simulink model "SPARCS_MIL"  (R2024a)
settings: Solver=VariableStepAuto  StartTime=0.0  StopTime=10.0  RelTol=1e-3
undefined symbols (not defined in the file or in its folder): attitude, epoch, IAU, juliandate, km, m, om0_x, om0_y, om0_z, s, satellite, simulator, WMM2020
libraries: simulink_extras x16, sharedtransform x14, SepehrMILLib x10, aerolibconvert2 x9, matrix_library x3, simulink x3, aerolibutil x3, vrlib x2, aerolibgravity2 x2, aerolibtransform2 x2
(part 2 of 2)

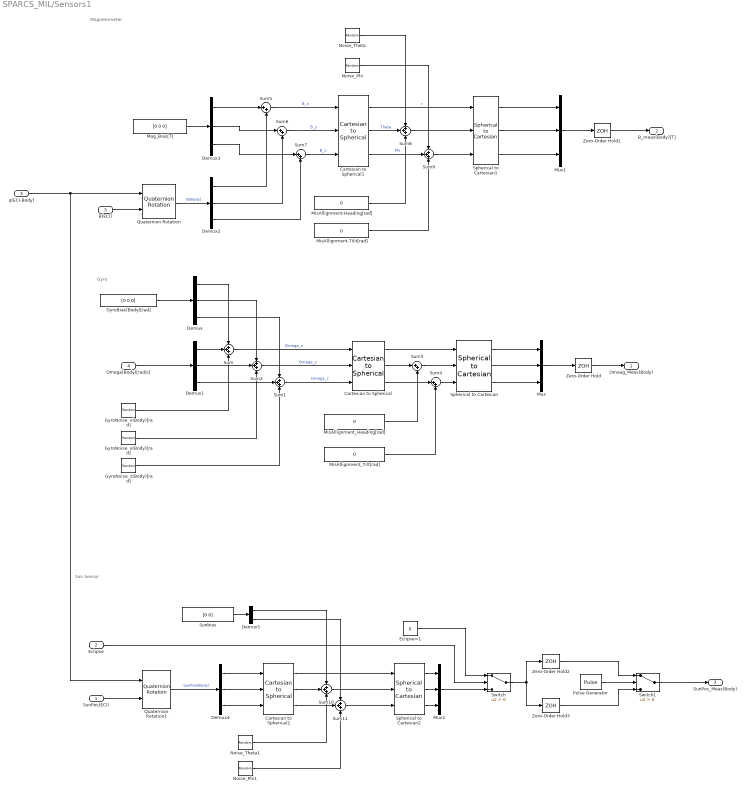
== system SPARCS_MIL/Sensors1 ==
  note: Magnetometer
  note: Sun Sensor
  note: Gyro
  SunPos(ECI) : Inport
  Eclipse : Inport  Port=2
  q(ECI-Body) : Inport  Port=3
  Omega(Body)[rad/s] : Inport  Port=4
  B(ECI) : InportShadow  Port=3
  Cartesian to Spherical : simulink_extras/Transformations/Cartesian to Spherical
  Cartesian to Spherical1 : simulink_extras/Transformations/Cartesian to Spherical
  Cartesian to Spherical2 : simulink_extras/Transformations/Cartesian to Spherical
  Demux{,1..4} (5 alike) : Demux  Outputs=3
  Demux5 : Demux  Outputs=2
  Eclipse=1 : Constant  Value=0
  GyroBias(Body)[rad] : Constant  Value=[0 0 0]
  GyroNoise_x(Body)[rad] : RandomNumber  SampleTime=0.1
  GyroNoise_y(Body)[rad] : RandomNumber  SampleTime=0.1
  GyroNoise_z(Body)[rad] : RandomNumber  SampleTime=0.1
  Mag_Bias[T] : Constant  Value=[0 0 0]
  MisAllignment-Heading[rad] : Constant  Value=0
  MisAllignment-Tilit[rad] : Constant  Value=0
  MisAllignment_Heading[rad] : Constant  Value=0
  MisAllignment_Tilt[rad] : Constant  Value=0
  Mux : Mux  Inputs=3
  Mux1 : Mux  Inputs=3
  Mux2 : Mux  Inputs=3
  Noise_Phi : RandomNumber  SampleTime=0.1
  Noise_Phi1 : RandomNumber  SampleTime=0.1
  Noise_Theta : RandomNumber  SampleTime=0.1
  Noise_Theta1 : RandomNumber  SampleTime=0.1
  Pulse Generator : DiscretePulseGenerator  Period=10  PulseWidth=5
  Quaternion Rotation : aerolibutil/Quaternion Rotation
  Quaternion Rotation1 : aerolibutil/Quaternion Rotation
  Spherical to Cartesian : simulink_extras/Transformations/Spherical to Cartesian
  Spherical to Cartesian1 : simulink_extras/Transformations/Spherical to Cartesian
  Spherical to Cartesian2 : simulink_extras/Transformations/Spherical to Cartesian
  Sum{,1..2,8..11} (7 alike) : Sum  Inputs=+++
  Sum{3..7} (5 alike) : Sum  Inputs=|++
  Sunbias : Constant  Value=[0 0]
  Switch : Switch  Criteria=u2 > Threshold  SaturateOnIntegerOverflow=off  InputSameDT=off
  Switch1 : Switch  Criteria=u2 > Threshold  SaturateOnIntegerOverflow=off  InputSameDT=off
  Zero-Order Hold{,1..3} (4 alike) : ZeroOrderHold  SampleTime=-1
  Omeag_Meas(Body) : Outport
  B_meas(Body)[T] : Outport  Port=2
  SunPos_Meas(Body) : Outport  Port=3
  wires:
  Spherical to Cartesian/1 -> Mux/1
  Demux1/1 -> Sum/2
  Cartesian to Spherical/2 -> Sum3/1
  Sum4/1 -> Spherical to Cartesian/3
  Demux/1 -> Sum/1
  Cartesian to Spherical/3 -> Sum4/1
  Sum1/1 -> Cartesian to Spherical/3  "Omega_z"
  Demux/3 -> Sum1/1
  Cartesian to Spherical/1 -> Spherical to Cartesian/1
  Spherical to Cartesian/2 -> Mux/2
  GyroNoise_y(Body)[rad]/1 -> Sum2/3
  GyroNoise_x(Body)[rad]/1 -> Sum/3
  Demux/2 -> Sum2/1
  GyroBias(Body)[rad]/1 -> Demux/1
  Demux1/2 -> Sum2/2
  Sum2/1 -> Cartesian to Spherical/2  "Omega_y"
  Sum/1 -> Cartesian to Spherical/1  "Omega_x"
  GyroNoise_z(Body)[rad]/1 -> Sum1/3
  Mux/1 -> Zero-Order Hold/1
  Sum3/1 -> Spherical to Cartesian/2
  Spherical to Cartesian/3 -> Mux/3
  MisAllignment_Tilt[rad]/1 -> Sum4/2
  MisAllignment_Heading[rad]/1 -> Sum3/2
  Omega(Body)[rad/s]/1 -> Demux1/1
  Zero-Order Hold/1 -> Omeag_Meas(Body)/1
  Demux1/3 -> Sum1/2
  Zero-Order Hold1/1 -> B_meas(Body)[T]/1
  Mux1/1 -> Zero-Order Hold1/1
  Spherical to Cartesian1/2 -> Mux1/2
  Demux2/3 -> Sum7/2
  Demux3/2 -> Sum6/1
  Quaternion Rotation/1 -> Demux2/1  "B(Body)"
  Cartesian to Spherical1/2 -> Sum8/2  "Theta"
  Demux2/1 -> Sum5/2
  Sum8/1 -> Spherical to Cartesian1/2
  Spherical to Cartesian1/3 -> Mux1/3
  MisAllignment-Heading[rad]/1 -> Sum8/3
  Sum9/1 -> Spherical to Cartesian1/3
  MisAllignment-Tilit[rad]/1 -> Sum9/3
  Noise_Theta/1 -> Sum8/1
  Spherical to Cartesian1/1 -> Mux1/1
  Mag_Bias[T]/1 -> Demux3/1
  Sum6/1 -> Cartesian to Spherical1/2  "B_y"
  Demux3/1 -> Sum5/1
  Cartesian to Spherical1/1 -> Spherical to Cartesian1/1  "r"
  Demux2/2 -> Sum6/2
  Cartesian to Spherical1/3 -> Sum9/2  "Phi"
  Demux3/3 -> Sum7/1
  Noise_Phi/1 -> Sum9/1
  Sum5/1 -> Cartesian to Spherical1/1  "B_x"
  Sum7/1 -> Cartesian to Spherical1/3  "B_z"
  q(ECI-Body)/1 -> Quaternion Rotation/1, Quaternion Rotation1/1
  B(ECI)/1 -> Quaternion Rotation/2
  Cartesian to Spherical2/1 -> Spherical to Cartesian2/1
  SunPos(ECI)/1 -> Quaternion Rotation1/2
  Switch1/1 -> SunPos_Meas(Body)/1
  Pulse Generator/1 -> Switch1/2
  Zero-Order Hold3/1 -> Switch1/3
  Zero-Order Hold2/1 -> Switch1/1
  Spherical to Cartesian2/2 -> Mux2/2
  Cartesian to Spherical2/2 -> Sum10/2
  Demux4/2 -> Cartesian to Spherical2/2
  Demux5/1 -> Sum10/1
  Switch/1 -> Zero-Order Hold2/1, Zero-Order Hold3/1
  Demux4/1 -> Cartesian to Spherical2/1
  Spherical to Cartesian2/3 -> Mux2/3
  Mux2/1 -> Switch/3
  Noise_Phi1/1 -> Sum11/3
  Eclipse/1 -> Switch/2
  Eclipse=1/1 -> Switch/1
  Spherical to Cartesian2/1 -> Mux2/1
  Sum10/1 -> Spherical to Cartesian2/2
  Sunbias/1 -> Demux5/1
  Quaternion Rotation1/1 -> Demux4/1  "SunPos(Body)"
  Noise_Theta1/1 -> Sum10/3
  Cartesian to Spherical2/3 -> Sum11/2
  Demux5/2 -> Sum11/1
  Demux4/3 -> Cartesian to Spherical2/3
  Sum11/1 -> Spherical to Cartesian2/3

== system SPARCS_MIL/Subsystem3 ==
  In1 : Inport
  In3 : Inport  Port=2
  If : If
  If Action Subsystem : Subsystem  TreatAsAtomicUnit=on
  If Action Subsystem1 : Subsystem  TreatAsAtomicUnit=on
  In2 : InportShadow
  Merge : Merge
  Out1 : Outport
  wires:
  If/2 -> If Action Subsystem/Action
  If/1 -> If Action Subsystem1/Action
  In1/1 -> If Action Subsystem1/1(In1)
  In2/1 -> If Action Subsystem/1(In1)
  If Action Subsystem/1(Out1) -> Merge/1
  If Action Subsystem1/1(Out1) -> Merge/2
  Merge/1 -> Out1/1
  In3/1 -> If/1

== system SPARCS_MIL/sensors sim ==
  In1 : Inport
  Out1 : Outport
  wires:
  In1/1 -> Out1/1

== system SPARCS_MIL/telecommand receiver ==
  In1 : Inport
  telecommand : Outport
  wires:
  In1/1 -> telecommand/1

== system SPARCS_MIL/telemetry transponder ==
  In1 : Inport
  telecommand : Outport
  wires:
  In1/1 -> telecommand/1

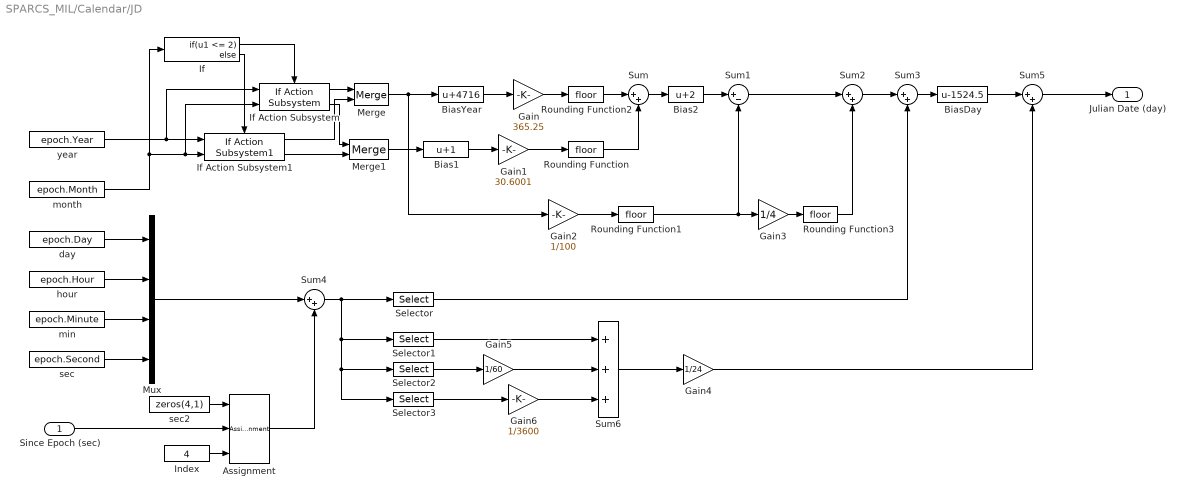
== system SPARCS_MIL/Calendar/JD ==
  Since Epoch (sec) : Inport  OutMin=0  PortDimensions=1
  Assignment : Assignment  IndexOptions=Index vector (port)  Indices=1  OutputSizes=1
  Bias1 : Bias  Bias=1  SaturateOnIntegerOverflow=off
  Bias2 : Bias  Bias=2  SaturateOnIntegerOverflow=off
  BiasDay : Bias  Bias=-1524.5  SaturateOnIntegerOverflow=off
  BiasYear : Bias  Bias=4716  SaturateOnIntegerOverflow=off
  Gain : Gain  Gain=365.25
  Gain1 : Gain  Gain=30.6001
  Gain2 : Gain  Gain=1/100
  Gain3 : Gain  Gain=1/4
  Gain4 : Gain  Gain=1/24
  Gain5 : Gain  Gain=1/60
  Gain6 : Gain  Gain=1/3600
  If : If  IfExpression=u1 <= 2
  If Action Subsystem : aerolibconvert2/Julian Date Conversion/If Action Subsystem  SystemSampleTime=-1  VariantActivationTime=update diagram  AllowFlexibleInterface=on  Latency=0  AutoFrameSizeCalculation=off
  If Action Subsystem1 : aerolibconvert2/Julian Date Conversion/If Action Subsystem1  SystemSampleTime=-1  VariantActivationTime=update diagram  AllowFlexibleInterface=on  Latency=0  AutoFrameSizeCalculation=off
  Index : Constant  Value=4
  Merge : Merge
  Merge1 : Merge
  Mux : Mux
  Rounding Function{,1..3} (4 alike) : Rounding
  Selector : Selector  InputPortWidth=4  IndexOptions=Index vector (dialog)  Indices=[1]  OutputSizes=1
  Selector1 : Selector  InputPortWidth=4  IndexOptions=Index vector (dialog)  Indices=[2]  OutputSizes=1
  Selector2 : Selector  InputPortWidth=4  IndexOptions=Index vector (dialog)  Indices=[3]  OutputSizes=1
  Selector3 : Selector  InputPortWidth=4  IndexOptions=Index vector (dialog)  Indices=[4]  OutputSizes=1
  Sum{,2..5} (5 alike) : Sum  Inputs=|++
  Sum1 : Sum  Inputs=|+-
  Sum6 : Sum  Inputs=+++
  day : Constant  Value=epoch.Day
  hour : Constant  Value=epoch.Hour
  min : Constant  Value=epoch.Minute
  month : Constant  Value=epoch.Month
  sec : Constant  Value=epoch.Second
  sec2 : Constant  Value=zeros(4,1)
  year : Constant  Value=epoch.Year
  Julian Date (day) : Outport  VectorParamsAs1DForOutWhenUnconnected=off
  wires:
  Merge1/1 -> Bias1/1
  Mux/1 -> Sum4/1
  month/1 -> If/1, If Action Subsystem1/2, If Action Subsystem/2
  Rounding Function/1 -> Sum/2
  day/1 -> Mux/1
  If Action Subsystem1/2 -> Merge1/2
  Sum/1 -> Bias2/1
  Sum6/1 -> Gain4/1
  BiasDay/1 -> Sum5/1
  hour/1 -> Mux/2
  Selector/1 -> Sum3/2
  sec/1 -> Mux/4
  Since Epoch (sec)/1 -> Assignment/2
  If/2 -> If Action Subsystem1/Action
  Rounding Function1/1 -> Sum1/2, Gain3/1
  Gain5/1 -> Sum6/2
  Assignment/1 -> Sum4/2
  Bias2/1 -> Sum1/1
  Gain/1 -> Rounding Function2/1
  Gain2/1 -> Rounding Function1/1
  Sum4/1 -> Selector/1, Selector3/1, Selector2/1, Selector1/1
  If Action Subsystem/1 -> Merge/1
  year/1 -> If Action Subsystem1/1, If Action Subsystem/1
  Gain6/1 -> Sum6/3
  Sum3/1 -> BiasDay/1
  If Action Subsystem/2 -> Merge1/1
  Bias1/1 -> Gain1/1
  Rounding Function3/1 -> Sum2/2
  Gain1/1 -> Rounding Function/1
  sec2/1 -> Assignment/1
  Sum1/1 -> Sum2/1
  Sum5/1 -> Julian Date (day)/1
  Selector1/1 -> Sum6/1
  Sum2/1 -> Sum3/1
  Gain4/1 -> Sum5/2
  BiasYear/1 -> Gain/1
  Merge/1 -> BiasYear/1, Gain2/1
  Gain3/1 -> Rounding Function3/1
  Selector2/1 -> Gain5/1
  Rounding Function2/1 -> Sum/1
  Selector3/1 -> Gain6/1
  If/1 -> If Action Subsystem/Action
  min/1 -> Mux/3
  If Action Subsystem1/1 -> Merge/2
  Index/1 -> Assignment/3

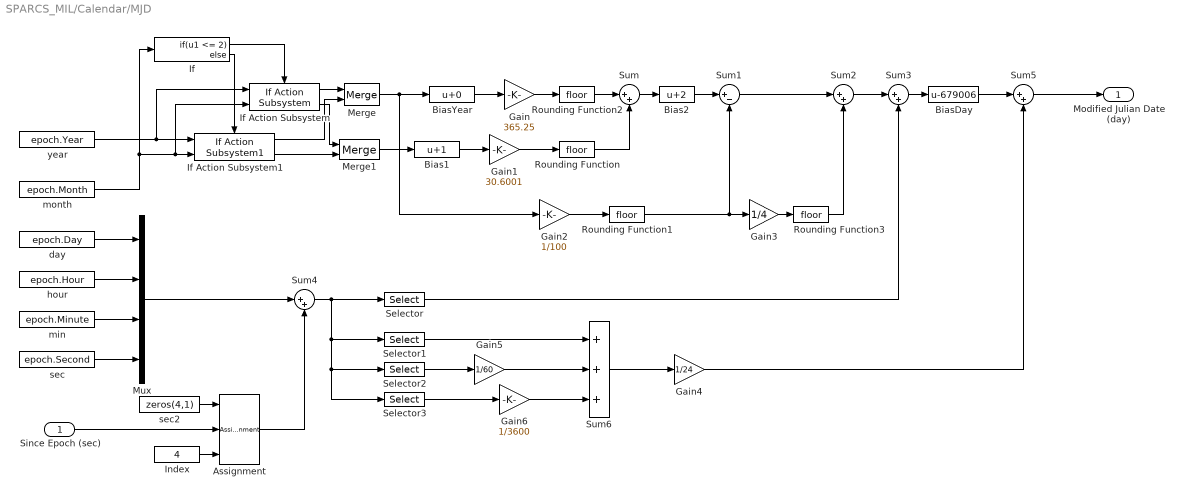
== system SPARCS_MIL/Calendar/MJD ==
  Since Epoch (sec) : Inport  OutMin=0  PortDimensions=1
  Assignment : Assignment  IndexOptions=Index vector (port)  Indices=1  OutputSizes=1
  Bias1 : Bias  Bias=1  SaturateOnIntegerOverflow=off
  Bias2 : Bias  Bias=2  SaturateOnIntegerOverflow=off
  BiasDay : Bias  Bias=-679006  SaturateOnIntegerOverflow=off
  BiasYear : Bias  SaturateOnIntegerOverflow=off
  Gain : Gain  Gain=365.25
  Gain1 : Gain  Gain=30.6001
  Gain2 : Gain  Gain=1/100
  Gain3 : Gain  Gain=1/4
  Gain4 : Gain  Gain=1/24
  Gain5 : Gain  Gain=1/60
  Gain6 : Gain  Gain=1/3600
  If : If  IfExpression=u1 <= 2
  If Action Subsystem : aerolibconvert2/Julian Date Conversion/If Action Subsystem  SystemSampleTime=-1  VariantActivationTime=update diagram  AllowFlexibleInterface=on  Latency=0  AutoFrameSizeCalculation=off
  If Action Subsystem1 : aerolibconvert2/Julian Date Conversion/If Action Subsystem1  SystemSampleTime=-1  VariantActivationTime=update diagram  AllowFlexibleInterface=on  Latency=0  AutoFrameSizeCalculation=off
  Index : Constant  Value=4
  Merge : Merge
  Merge1 : Merge
  Mux : Mux
  Rounding Function{,1..3} (4 alike) : Rounding
  Selector : Selector  InputPortWidth=4  IndexOptions=Index vector (dialog)  Indices=[1]  OutputSizes=1
  Selector1 : Selector  InputPortWidth=4  IndexOptions=Index vector (dialog)  Indices=[2]  OutputSizes=1
  Selector2 : Selector  InputPortWidth=4  IndexOptions=Index vector (dialog)  Indices=[3]  OutputSizes=1
  Selector3 : Selector  InputPortWidth=4  IndexOptions=Index vector (dialog)  Indices=[4]  OutputSizes=1
  Sum{,2..5} (5 alike) : Sum  Inputs=|++
  Sum1 : Sum  Inputs=|+-
  Sum6 : Sum  Inputs=+++
  day : Constant  Value=epoch.Day
  hour : Constant  Value=epoch.Hour
  min : Constant  Value=epoch.Minute
  month : Constant  Value=epoch.Month
  sec : Constant  Value=epoch.Second
  sec2 : Constant  Value=zeros(4,1)
  year : Constant  Value=epoch.Year
  Modified Julian Date (day) : Outport  VectorParamsAs1DForOutWhenUnconnected=off
  wires:
  Rounding Function/1 -> Sum/2
  If/2 -> If Action Subsystem1/Action
  Gain4/1 -> Sum5/2
  BiasYear/1 -> Gain/1
  Bias2/1 -> Sum1/1
  Selector1/1 -> Sum6/1
  Sum/1 -> Bias2/1
  Sum2/1 -> Sum3/1
  BiasDay/1 -> Sum5/1
  Selector/1 -> Sum3/2
  Sum1/1 -> Sum2/1
  year/1 -> If Action Subsystem1/1, If Action Subsystem/1
  Sum5/1 -> Modified Julian Date (day)/1
  Sum6/1 -> Gain4/1
  hour/1 -> Mux/2
  Gain/1 -> Rounding Function2/1
  Merge1/1 -> Bias1/1
  Since Epoch (sec)/1 -> Assignment/2
  Gain6/1 -> Sum6/3
  Gain2/1 -> Rounding Function1/1
  Mux/1 -> Sum4/1
  Rounding Function1/1 -> Sum1/2, Gain3/1
  Rounding Function3/1 -> Sum2/2
  Sum3/1 -> BiasDay/1
  Selector3/1 -> Gain6/1
  Rounding Function2/1 -> Sum/1
  Gain1/1 -> Rounding Function/1
  sec2/1 -> Assignment/1
  day/1 -> Mux/1
  Bias1/1 -> Gain1/1
  min/1 -> Mux/3
  Gain3/1 -> Rounding Function3/1
  If/1 -> If Action Subsystem/Action
  Gain5/1 -> Sum6/2
  If Action Subsystem1/1 -> Merge/2
  Sum4/1 -> Selector/1, Selector3/1, Selector2/1, Selector1/1
  Merge/1 -> BiasYear/1, Gain2/1
  If Action Subsystem/1 -> Merge/1
  Selector2/1 -> Gain5/1
  If Action Subsystem/2 -> Merge1/1
  month/1 -> If/1, If Action Subsystem1/2, If Action Subsystem/2
  sec/1 -> Mux/4
  If Action Subsystem1/2 -> Merge1/2
  Assignment/1 -> Sum4/2
  Index/1 -> Assignment/3

== system SPARCS_MIL/Kinematics and Dynamics/Dynamics ==
  T_body : Inport
  I : Inport  Port=2
  om0 : Inport  Port=3
  Add : Sum
  Add1 : Sum
  Add2 : Sum
  Demux : Demux  Outputs=3
  Demux1 : Demux  Outputs=3
  Demux2 : Demux  Outputs=3
  Divide : Product  Inputs=*/
  Integrator : Integrator  InitialConditionSource=external  InitialCondition=om0_x
  Integrator1 : Integrator  InitialConditionSource=external  InitialCondition=om0_y
  Integrator2 : Integrator  InitialConditionSource=external  InitialCondition=om0_z
  Mux : Mux  Inputs=3
  Product : Product
  Product1 : Product
  Product2 : Product
  gain_x : Subsystem
  gain_y : Subsystem
  gain_z : Subsystem
  om : Outport
  wires:
  Add1/1 -> Integrator2/1
  T_body/1 -> Divide/1
  Add2/1 -> Integrator1/1
  Integrator2/1 -> Mux/3, Product/2, Product1/2  "om_z"
  Add/1 -> Integrator/1
  Product2/1 -> gain_z/1(In_Gain_z)
  gain_z/1(Out_Gain_z) -> Add1/1
  Demux/1 -> Add/2
  Integrator/1 -> Product2/2, Product1/1, Mux/1  "om_x"
  Integrator1/1 -> Mux/2, Product/1, Product2/1  "om_y"
  I/1 -> Demux2/1, Divide/2
  gain_x/1(Out_Gain_x) -> Add/1
  Product1/1 -> gain_y/4(In_Gain_y)
  gain_y/1(Out_Gain_y) -> Add2/1
  Divide/1 -> Demux/1
  Product/1 -> gain_x/1(In_Gain_x)
  Demux/2 -> Add2/2
  Demux/3 -> Add1/2
  Mux/1 -> om/1
  om0/1 -> Demux1/1
  Demux1/1 -> Integrator/2
  Demux1/2 -> Integrator1/2
  Demux1/3 -> Integrator2/2
  Demux2/1 -> gain_z/2(I_x), gain_x/2(I_x), gain_y/1(I_x)
  Demux2/2 -> gain_y/2(I_y), gain_x/3(I_y), gain_z/3(I_y)
  Demux2/3 -> gain_x/4(I_z), gain_y/3(I_z), gain_z/4(I_z)

== system SPARCS_MIL/Kinematics and Dynamics/kinematics ==
  om : Inport
  Out1 : Outport
  wires:
  om/1 -> Out1/1

== system SPARCS_MIL/OBC/running.nominal.detum.detumb_soft/ADCS ==
  In1 : Inport
  ADCS : ModelReference  SimulationMode=Normal
  Model : ModelReference  SimulationMode=Normal

== system SPARCS_MIL/OBC/running.nominal.detum.detumb_soft/Telecommand digest ==
  telecommand : Inport
  Telecommand digest : ModelReference  SimulationMode=Normal
  Out1 : Outport
  Out2 : Outport  Port=2

== system SPARCS_MIL/OBC/running.nominal.detum.detumb_soft/power ==
  In1 : Inport
  ADCS : ModelReference  SimulationMode=Normal
  Model : ModelReference  SimulationMode=Normal

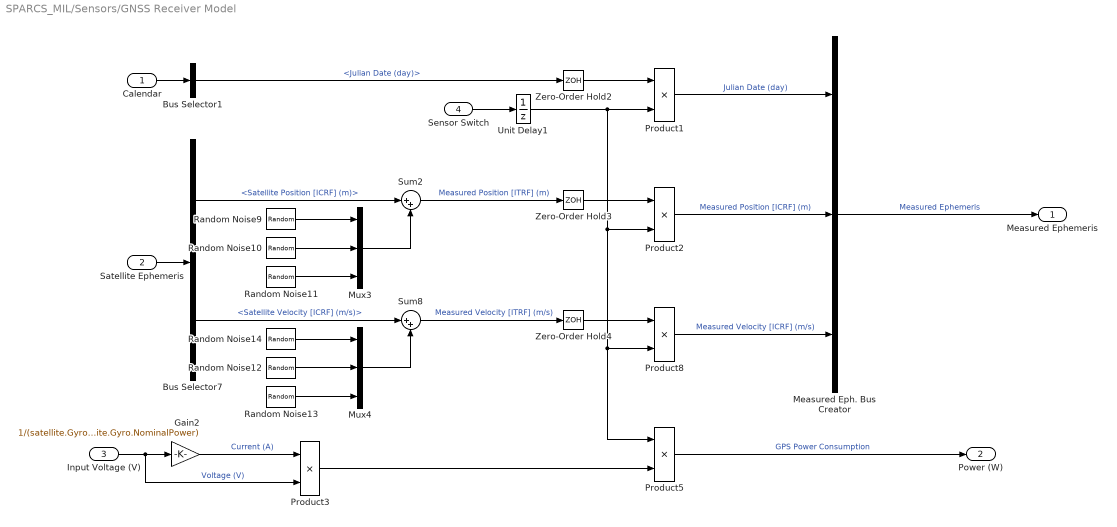
== system SPARCS_MIL/Sensors/GNSS Receiver Model ==
  Calendar : Inport
  Satellite Ephemeris : Inport  Port=2
  Input Voltage (V) : Inport  Port=3
  Sensor Switch : Inport  Port=4
  Bus Selector1 : BusSelector  OutputSignals=Julian Date (day)
  Bus Selector7 : BusSelector  OutputSignals=Satellite Position [ICRF] (m),Satellite Velocity [ICRF] (m/s)
  Gain2 : Gain  Gain=1/(satellite.Gyro.NominalVoltage^2/satellite.Gyro.NominalPower)
  Measured Eph. Bus Creator : BusCreator  Inputs=3
  Mux3 : Mux  Inputs=3
  Mux4 : Mux  Inputs=3
  Product{1..3,5,8} (5 alike) : Product
  Random Noise10 : RandomNumber  Mean=satellite.GPS.Position.Bias  Variance=satellite.GPS.Position.NoiseSTDDEV^2  SampleTime=1/satellite.GPS.Frequency
  Random Noise11 : RandomNumber  Mean=satellite.GPS.Position.Bias  Variance=satellite.GPS.Position.NoiseSTDDEV^2  SampleTime=1/satellite.GPS.Frequency
  Random Noise12 : RandomNumber  Mean=satellite.GPS.Velocity.Bias  Variance=satellite.GPS.Position.NoiseSTDDEV^2  SampleTime=1/satellite.GPS.Frequency
  Random Noise13 : RandomNumber  Mean=satellite.GPS.Velocity.Bias  Variance=satellite.GPS.Position.NoiseSTDDEV^2  SampleTime=1/satellite.GPS.Frequency
  Random Noise14 : RandomNumber  Mean=satellite.GPS.Velocity.Bias  Variance=satellite.GPS.Position.NoiseSTDDEV^2  SampleTime=1/satellite.GPS.Frequency
  Random Noise9 : RandomNumber  Mean=satellite.GPS.Position.Bias  Variance=satellite.GPS.Position.NoiseSTDDEV^2  SampleTime=1/satellite.GPS.Frequency
  Sum2 : Sum  Inputs=|++
  Sum8 : Sum  Inputs=|++
  Unit Delay1 : UnitDelay  SampleTime=-1  HasFrameUpgradeWarning=on
  Zero-Order Hold2 : ZeroOrderHold  SampleTime=1/satellite.GPS.Frequency
  Zero-Order Hold3 : ZeroOrderHold  SampleTime=1/satellite.GPS.Frequency
  Zero-Order Hold4 : ZeroOrderHold  SampleTime=1/satellite.GPS.Frequency
  Measured Ephemeris : Outport
  Power (W) : Outport  Port=2
  wires:
  Product1/1 -> Measured Eph. Bus Creator/1  "Julian Date (day)"
  Random Noise12/1 -> Mux4/2
  Sum8/1 -> Zero-Order Hold4/1  "Measured Velocity [ITRF] (m/s)"
  Sensor Switch/1 -> Unit Delay1/1
  Zero-Order Hold3/1 -> Product2/1
  Product8/1 -> Measured Eph. Bus Creator/3  "Measured Velocity [ICRF] (m/s)"
  Measured Eph. Bus Creator/1 -> Measured Ephemeris/1  "Measured Ephemeris"
  Zero-Order Hold2/1 -> Product1/1
  Unit Delay1/1 -> Product1/2, Product2/2, Product8/2, Product5/1
  Product2/1 -> Measured Eph. Bus Creator/2  "Measured Position [ICRF] (m)"
  Product3/1 -> Product5/2
  Product5/1 -> Power (W)/1  "GPS Power Consumption"
  Random Noise9/1 -> Mux3/1
  Bus Selector7/2 -> Sum8/1  "<Satellite Velocity [ICRF] (m/s)>"
  Zero-Order Hold4/1 -> Product8/1
  Bus Selector7/1 -> Sum2/1  "<Satellite Position [ICRF] (m)>"
  Input Voltage (V)/1 -> Gain2/1, Product3/2  "Voltage (V)"
  Sum2/1 -> Zero-Order Hold3/1  "Measured Position [ITRF] (m)"
  Mux3/1 -> Sum2/2
  Random Noise10/1 -> Mux3/2
  Mux4/1 -> Sum8/2
  Random Noise11/1 -> Mux3/3
  Random Noise13/1 -> Mux4/3
  Bus Selector1/1 -> Zero-Order Hold2/1  "<Julian Date (day)>"
  Satellite Ephemeris/1 -> Bus Selector7/1
  Calendar/1 -> Bus Selector1/1
  Gain2/1 -> Product3/1  "Current (A)"
  Random Noise14/1 -> Mux4/1

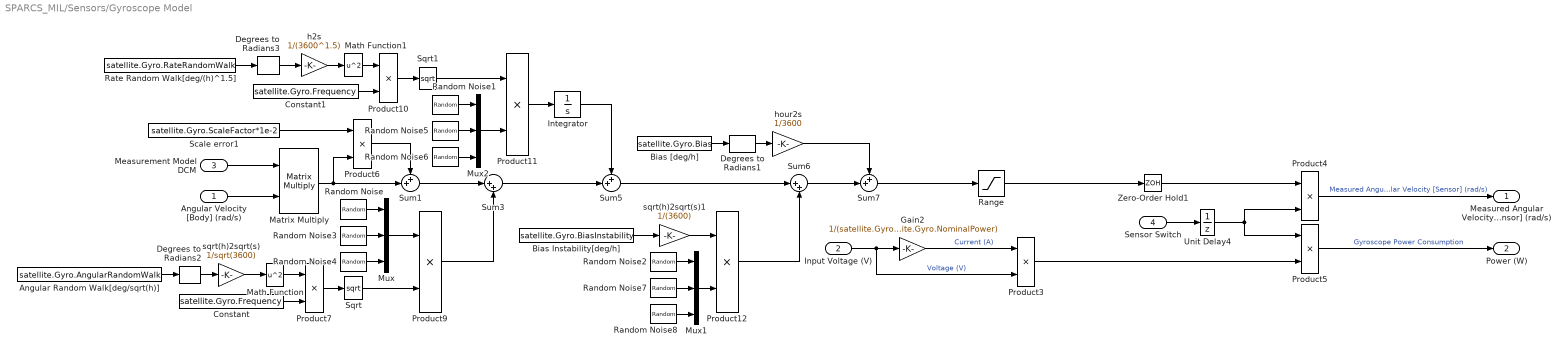
== system SPARCS_MIL/Sensors/Gyroscope Model ==
  Angular Velocity [Body] (rad/s) : Inport
  Input Voltage (V) : Inport  Port=2
  Measurement Model DCM : Inport  Port=3
  Sensor Switch : Inport  Port=4
  Angular Random Walk[deg/sqrt(h)] : Constant  Value=satellite.Gyro.AngularRandomWalk
  Bias Instability[deg/h] : Constant  Value=satellite.Gyro.BiasInstability
  Bias [deg/h] : Constant  Value=satellite.Gyro.Bias
  Constant : Constant  Value=satellite.Gyro.Frequency
  Constant1 : Constant  Value=satellite.Gyro.Frequency
  Degrees to Radians1 : simulink_extras/Transformations/Degrees to Radians
  Degrees to Radians2 : simulink_extras/Transformations/Degrees to Radians
  Degrees to Radians3 : simulink_extras/Transformations/Degrees to Radians
  Gain2 : Gain  Gain=1/(satellite.Gyro.NominalVoltage^2/satellite.Gyro.NominalPower)
  Integrator : Integrator  InitialCondition=[0;0;0]
  Math Function : Math  Operator=square  SignedPower=on
  Math Function1 : Math  Operator=square  SignedPower=on
  Matrix Multiply : Product  Multiplication=Matrix(*)
  Mux : Mux  Inputs=3
  Mux1 : Mux  Inputs=3
  Mux2 : Mux  Inputs=3
  Product{3..7,9..12} (9 alike) : Product
  Random Noise{,1..8} (9 alike) : RandomNumber  SampleTime=1/satellite.Gyro.Frequency
  Range : Saturate  UpperLimit=satellite.Gyro.Range(2)  LowerLimit=satellite.Gyro.Range(1)
  Rate Random Walk[deg/(h)^1.5] : Constant  Value=satellite.Gyro.RateRandomWalk
  Scale error1 : Constant  Value=satellite.Gyro.ScaleFactor*1e-2
  Sqrt : Sqrt
  Sqrt1 : Sqrt
  Sum1 : Sum  Inputs=++|
  Sum3 : Sum  Inputs=|++
  Sum5 : Sum  Inputs=++|
  Sum6 : Sum  Inputs=|++
  Sum7 : Sum  Inputs=++|
  Unit Delay4 : UnitDelay  SampleTime=-1  HasFrameUpgradeWarning=on
  Zero-Order Hold1 : ZeroOrderHold  SampleTime=1/satellite.Gyro.Frequency
  h2s : Gain  Gain=1/(3600^1.5)
  hour2s : Gain  Gain=1/3600
  sqrt(h)2sqrt(s) : Gain  Gain=1/sqrt(3600)
  sqrt(h)2sqrt(s)1 : Gain  Gain=1/(3600)
  Measured Angular Velocity [Sensor] (rad/s) : Outport  PortDimensions=[3,1]
  Power (W) : Outport  Port=2
  wires:
  Sqrt/1 -> Product9/2
  Sum1/1 -> Sum3/1
  Sum6/1 -> Sum7/2
  hour2s/1 -> Sum7/1
  Matrix Multiply/1 -> Product6/2, Sum1/2
  Range/1 -> Zero-Order Hold1/1
  Random Noise3/1 -> Mux/2
  Mux/1 -> Product9/1
  Degrees to Radians3/1 -> h2s/1
  Product12/1 -> Sum6/2
  Product9/1 -> Sum3/2
  Product10/1 -> Sqrt1/1
  Random Noise5/1 -> Mux2/2
  Sum5/1 -> Sum6/1
  Integrator/1 -> Sum5/1
  Random Noise6/1 -> Mux2/3
  Math Function/1 -> Product7/1
  Random Noise7/1 -> Mux1/2
  sqrt(h)2sqrt(s)/1 -> Math Function/1
  Mux2/1 -> Product11/2
  Sum7/1 -> Range/1
  Angular Velocity [Body] (rad/s)/1 -> Matrix Multiply/2
  Product3/1 -> Product5/2
  Random Noise2/1 -> Mux1/1
  Constant/1 -> Product7/2
  Bias Instability[deg/h]/1 -> sqrt(h)2sqrt(s)1/1
  Random Noise4/1 -> Mux/3
  Angular Random Walk[deg/sqrt(h)]/1 -> Degrees to Radians2/1
  Gain2/1 -> Product3/1  "Current (A)"
  Random Noise/1 -> Mux/1
  Rate Random Walk[deg/(h)^1.5]/1 -> Degrees to Radians3/1
  Measurement Model DCM/1 -> Matrix Multiply/1
  Product6/1 -> Sum1/1
  Math Function1/1 -> Product10/1
  h2s/1 -> Math Function1/1
  Constant1/1 -> Product10/2
  Product7/1 -> Sqrt/1
  Scale error1/1 -> Product6/1
  Zero-Order Hold1/1 -> Product4/1
  Mux1/1 -> Product12/2
  Sqrt1/1 -> Product11/1
  Product11/1 -> Integrator/1
  Sum3/1 -> Sum5/2
  Sensor Switch/1 -> Unit Delay4/1
  sqrt(h)2sqrt(s)1/1 -> Product12/1
  Bias [deg/h]/1 -> Degrees to Radians1/1
  Degrees to Radians2/1 -> sqrt(h)2sqrt(s)/1
  Product4/1 -> Measured Angular Velocity [Sensor] (rad/s)/1  "Measured Angular Velocity [Sensor] (rad/s)"
  Degrees to Radians1/1 -> hour2s/1
  Random Noise1/1 -> Mux2/1
  Input Voltage (V)/1 -> Product3/2, Gain2/1  "Voltage (V)"
  Unit Delay4/1 -> Product5/1, Product4/2
  Product5/1 -> Power (W)/1  "Gyroscope Power Consumption"
  Random Noise8/1 -> Mux1/3

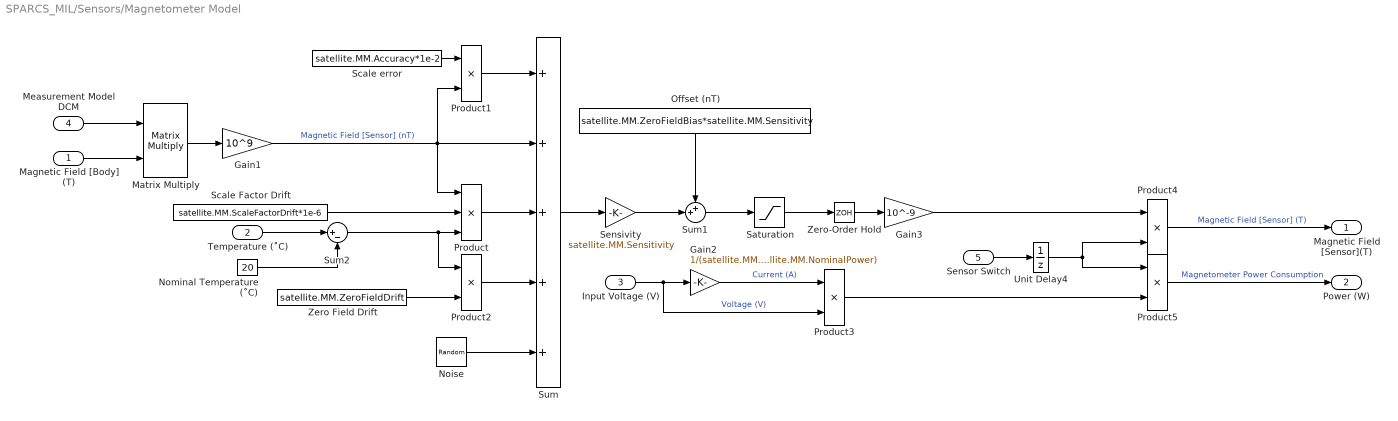
== system SPARCS_MIL/Sensors/Magnetometer Model ==
  Magnetic Field [Body] (T) : Inport
  Temperature (˚C) : Inport  Port=2
  Input Voltage (V) : Inport  Port=3
  Measurement Model DCM : Inport  Port=4
  Sensor Switch : Inport  Port=5
  Gain1 : Gain  Gain=10^9
  Gain2 : Gain  Gain=1/(satellite.MM.NominalVoltage^2/satellite.MM.NominalPower)
  Gain3 : Gain  Gain=10^-9
  Matrix Multiply : Product  Multiplication=Matrix(*)
  Noise : RandomNumber  Variance=satellite.MM.NoiseVariance  SampleTime=1/satellite.MM.Frequency
  Nominal Temperature (˚C) : Constant  Value=20
  Offset (nT) : Constant  Value=satellite.MM.ZeroFieldBias*satellite.MM.Sensitivity
  Product : Product  Inputs=3
  Product{1..5} (5 alike) : Product
  Saturation : Saturate  UpperLimit=satellite.MM.Range(2)  LowerLimit=satellite.MM.Range(1)
  Scale Factor Drift : Constant  Value=satellite.MM.ScaleFactorDrift*1e-6
  Scale error : Constant  Value=satellite.MM.Accuracy*1e-2
  Sensivity : Gain  Gain=satellite.MM.Sensitivity
  Sum : Sum  Inputs=+++++
  Sum1 : Sum  Inputs=++|
  Sum2 : Sum  Inputs=|+-
  Unit Delay4 : UnitDelay  SampleTime=-1  HasFrameUpgradeWarning=on
  Zero Field Drift : Constant  Value=satellite.MM.ZeroFieldDrift
  Zero-Order Hold : ZeroOrderHold  SampleTime=1/satellite.MM.Frequency
  Magnetic Field [Sensor](T) : Outport  PortDimensions=[3,1]
  Power (W) : Outport  Port=2
  wires:
  Product3/1 -> Product5/2
  Scale error/1 -> Product1/1
  Sum2/1 -> Product/3, Product2/1
  Saturation/1 -> Zero-Order Hold/1
  Product2/1 -> Sum/4
  Zero-Order Hold/1 -> Gain3/1
  Nominal Temperature (˚C)/1 -> Sum2/2
  Gain2/1 -> Product3/1  "Current (A)"
  Offset (nT)/1 -> Sum1/1
  Measurement Model DCM/1 -> Matrix Multiply/1
  Temperature (˚C)/1 -> Sum2/1
  Product/1 -> Sum/3
  Product1/1 -> Sum/1
  Sensor Switch/1 -> Unit Delay4/1
  Input Voltage (V)/1 -> Gain2/1, Product3/2  "Voltage (V)"
  Sum/1 -> Sensivity/1
  Zero Field Drift/1 -> Product2/2
  Product4/1 -> Magnetic Field [Sensor](T)/1  "Magnetic Field [Sensor] (T)"
  Scale Factor Drift/1 -> Product/2
  Noise/1 -> Sum/5
  Gain1/1 -> Product1/2, Product/1, Sum/2  "Magnetic Field [Sensor] (nT)"
  Sum1/1 -> Saturation/1
  Sensivity/1 -> Sum1/2
  Magnetic Field [Body] (T)/1 -> Matrix Multiply/2
  Gain3/1 -> Product4/1
  Unit Delay4/1 -> Product4/2, Product5/1
  Matrix Multiply/1 -> Gain1/1
  Product5/1 -> Power (W)/1  "Magnetometer Power Consumption"

== system SPARCS_MIL/Sensors/Sun Sensor Model ==
  Eclipse : Inport
  q[ICRFtoBody] : Inport  Port=2
  SunPos[ICRF] : Inport  Port=3
  Cartesian to Spherical2 : simulink_extras/Transformations/Cartesian to Spherical
  Demux4 : Demux  Outputs=3
  Demux5 : Demux  Outputs=2
  Eclipse=1 : Constant  Value=0
  Mux2 : Mux  Inputs=3
  Noise_Phi1 : RandomNumber  SampleTime=0.1
  Noise_Theta1 : RandomNumber  SampleTime=0.1
  Pulse Generator1 : DiscretePulseGenerator  Period=10  PulseWidth=5
  Quaternion Rotation1 : aerolibutil/Quaternion Rotation
  Spherical to Cartesian2 : simulink_extras/Transformations/Spherical to Cartesian
  Sum10 : Sum  Inputs=+++
  Sum11 : Sum  Inputs=+++
  SunBias : Constant  Value=[0 0]
  Switch : Switch  Criteria=u2 > Threshold  SaturateOnIntegerOverflow=off  InputSameDT=off
  Switch2 : Switch  Criteria=u2 > Threshold  SaturateOnIntegerOverflow=off  InputSameDT=off
  Zero-Order Hold2 : ZeroOrderHold  SampleTime=-1
  Zero-Order Hold3 : ZeroOrderHold  SampleTime=-1
  SunPos_Meas[Body] : Outport
  wires:
  Switch2/1 -> SunPos_Meas[Body]/1
  Noise_Theta1/1 -> Sum10/3
  Spherical to Cartesian2/3 -> Mux2/3
  Demux4/1 -> Cartesian to Spherical2/1
  Spherical to Cartesian2/2 -> Mux2/2
  Demux5/1 -> Sum10/1
  Zero-Order Hold2/1 -> Switch2/1
  Cartesian to Spherical2/1 -> Spherical to Cartesian2/1
  Demux4/2 -> Cartesian to Spherical2/2
  Eclipse=1/1 -> Switch/1
  Spherical to Cartesian2/1 -> Mux2/1
  Mux2/1 -> Switch/3
  Demux5/2 -> Sum11/1
  Sum10/1 -> Spherical to Cartesian2/2
  Sum11/1 -> Spherical to Cartesian2/3
  Cartesian to Spherical2/2 -> Sum10/2
  Noise_Phi1/1 -> Sum11/3
  Demux4/3 -> Cartesian to Spherical2/3
  Pulse Generator1/1 -> Switch2/2
  SunPos[ICRF]/1 -> Quaternion Rotation1/2
  Eclipse/1 -> Switch/2
  Zero-Order Hold3/1 -> Switch2/3
  Switch/1 -> Zero-Order Hold2/1, Zero-Order Hold3/1
  Cartesian to Spherical2/3 -> Sum11/2
  Quaternion Rotation1/1 -> Demux4/1  "SunPos[Body]"
  SunBias/1 -> Demux5/1
  q[ICRFtoBody]/1 -> Quaternion Rotation1/1

== system SPARCS_MIL/Subsystem3/If Action Subsystem ==
  In1 : Inport
  Action Port : ActionPort  ActionPortLabel=else
  Out1 : Outport
  wires:
  In1/1 -> Out1/1

== system SPARCS_MIL/Subsystem3/If Action Subsystem1 ==
  In1 : Inport
  Action Port : ActionPort  ActionPortLabel=if(u1 > 0)
  Out1 : Outport
  wires:
  In1/1 -> Out1/1

== system SPARCS_MIL/Kinematics and Dynamics/Dynamics/gain_x ==
  In_Gain_x : Inport
  I_x : Inport  Port=2
  I_y : Inport  Port=3
  I_z : Inport  Port=4
  Divide : Product  Inputs=*/
  Product : Product
  Sum : Sum  Inputs=|-+
  Out_Gain_x : Outport
  wires:
  I_x/1 -> Divide/2
  I_z/1 -> Sum/2
  I_y/1 -> Sum/1
  Sum/1 -> Divide/1
  Divide/1 -> Product/2
  Product/1 -> Out_Gain_x/1
  In_Gain_x/1 -> Product/1

== system SPARCS_MIL/Kinematics and Dynamics/Dynamics/gain_y ==
  I_x : Inport
  I_y : Inport  Port=2
  I_z : Inport  Port=3
  In_Gain_y : Inport  Port=4
  Divide : Product  Inputs=*/
  Product : Product
  Sum : Sum  Inputs=|-+
  Out_Gain_y : Outport
  wires:
  Divide/1 -> Product/2
  Sum/1 -> Divide/1
  I_y/1 -> Divide/2
  I_x/1 -> Sum/1
  I_z/1 -> Sum/2
  In_Gain_y/1 -> Product/1
  Product/1 -> Out_Gain_y/1

== system SPARCS_MIL/Kinematics and Dynamics/Dynamics/gain_z ==
  In_Gain_z : Inport
  I_x : Inport  Port=2
  I_y : Inport  Port=3
  I_z : Inport  Port=4
  Divide : Product  Inputs=*/
  Product : Product
  Sum : Sum  Inputs=|-+
  Out_Gain_z : Outport
  wires:
  Divide/1 -> Product/2
  Sum/1 -> Divide/1
  I_y/1 -> Sum/1
  I_x/1 -> Sum/2
  I_z/1 -> Divide/2
  In_Gain_z/1 -> Product/1
  Product/1 -> Out_Gain_z/1

== matlab function SPARCS_MIL/Attitude Determination and Estimation Algorithms/MATLAB Function1 ==
  data: SunPos_ECI input; quat_TRIAD output; MagField_ECI input; SunPos_Body input; MagField_Body input; CovarianceMatrix output; RotationMatrix output; NoiseStd input; signQuat input
function [quat_TRIAD, CovarianceMatrix, RotationMatrix] = TRIAD(SunPos_ECI, MagField_ECI, SunPos_Body, MagField_Body, NoiseStd, signQuat)
% TRIAD Algorithm for Attitude Determination
% Inputs:
% - SunPos_ECI: Sun position vector in the inertial frame (ECI)
% - MagField_ECI: Magnetic field vector in the inertial frame (ECI)
% - SunPos_Body: Sun position vector in the body (spacecraft) frame
% - MagField_Body: Magnetic field vector in the body (spacecraft) frame
% - NoiseStd: [sigma1, sigma2] standard deviations of measurement noise
% - signQuat: sign parameter for quaternion calculation (e.g., ±1)
%
% Outputs:
% - quat_TRIAD: Quaternion representing the body-to-inertial rotation
% - CovarianceMatrix: Covariance matrix for the attitude estimation
% - RotationMatrix: Direction Cosine Matrix (DCM) from body to inertial frame

% Separate the noise standard deviations for more accurate and less accurate measurements
sigma_Sun = NoiseStd(1); % Standard deviation for Sun position measurement
sigma_Mag = NoiseStd(2); % Standard deviation for magnetic field measurement

% Reference Frame TRIAD Vectors (in ECI)
ref1 = SunPos_ECI;    % First vector (higher accuracy) in inertial frame
ref2 = cross(SunPos_ECI, MagField_ECI) / norm(cross(SunPos_ECI, MagField_ECI));
ref3 = cross(SunPos_ECI, ref2);  % Complete orthogonal basis

RefFrameMatrix = [ref1, ref2, ref3]; % TRIAD frame in terms of ECI vectors

% Body Frame TRIAD Vectors (in Spacecraft Frame)
body1 = SunPos_Body;  % First vector (higher accuracy) in body frame
body2 = cross(SunPos_Body, MagField_Body) / norm(cross(SunPos_Body, MagField_Body));
body3 = cross(SunPos_Body, body2); % Complete orthogonal basis

BodyFrameMatrix = [body1, body2, body3]; % TRIAD frame in terms of body vectors

% Estimated Rotation Matrix (DCM) from Body to Inertial Frame
RotationMatrix = RefFrameMatrix * BodyFrameMatrix';
RotationMatrix = transpose(RotationMatrix); % Transpose if convention requires it

% Convert Rotation Matrix to Quaternion
quat_TRIAD = DCMtoQuaternion(RotationMatrix, signQuat);

% Covariance Matrix Calculation for TRIAD
CovarianceMatrix = (sigma_Sun^2 * eye(3)) + ...
    (((sigma_Mag^2 - sigma_Sun^2) * (body1 * body1')) + ...
    (sigma_Sun^2 * (dot(body1, body2) * ((body1 * body2') + (body2 * body1'))))) / ...
    (norm(cross(body1, body2))^2));

end

== matlab function SPARCS_MIL/Attitude Determination and Estimation Algorithms/MATLAB Function ==
  data: r input; q_TRIAD output; b input; sigma input; sgn input; Cov output; A_est output
function [q_TRIAD, Cov, A_est] = TRIAD(r,b, sigma, sgn)
% Algorithm is written by
%  Markley, F. L., “Attitude Determination Using Two Vector Measurements,” 1998

r1 = r(:,1); %More accuarate measurement in reference frame
r2 = r(:,2); %Less accuarate measurement in reference frame

b1 = b(:,1); %More accuarate measurement in body frame
b2 = b(:,2); %Less accuarate measurement in body frame

sigma1 = sigma(1,:); %More accuarate measurement standart deviation
sigma2 = sigma(2,:); %Less accuarate

v1 = r1;    %1st component of TRIAD in reference frame
v2 = cross(r1, r2) / norm(cross(r1 , r2));
v3 = cross(r1, v2);
v = [v1 v2 v3]; %TRIAD frame in terms of reference vectors

w1 = b1;    %1st component of TRIAD in body frame
w2 = cross(b1 , b2) / norm(cross(b1 , b2));
w3 = cross(b1, w2);
w = [w1 w2 w3]; %TRIAD frame in terms of observation vectors in body

A_est = v * w'; %Estimated Attitude Matrix with TRIAD
A_est = transpose(A_est);
q_TRIAD =  Ctoq(A_est, sgn);

%COVARIANCE MATRIX of TRIAD 
% Shuster, M. D., and Oh, S. D., “Three-axis attitude determination from vector observations,” Journal of Guidance and Control,
% Vol. 4, No. 1, 1981, pp. 70–77. https://doi.org/10.2514/3.19717.

Cov = (sigma1^2 * eye(3)) + ...
    ((((sigma2^2 - sigma1^2) * (b1 * b1')) + ...
    (sigma1^2 * (dot(b1, b2) * ((b1* b2') + (b2 * b1'))))) / ...
    ((norm(cross(b1, b2)))^2));

end

== stateflow chart SPARCS_MIL/OBC ==
  state boot
    state ?
    (default) -> ?
  state running
    state nominal
      state detum
        state detumb_soft
        (default) -> detumb_soft
      state point
      point -> ?
      (default) -> ? [order 1]
      (default) -> point [order 1]
    state safe
    (default) -> nominal
    safe -> nominal
    nominal -> safe
  (default) -> boot
  boot -> running
  data: sf_internal_action_state_placeholder_data local double size=1 =0; sf_internal_action_state_placeholder_data local double size=1 =0; sensors input; telecommand input; telemetry output
